simulink model "barometer"  (R2018a)
settings: Solver=VariableStepAuto  StartTime=0.0  StopTime=10.0  RelTol=1e-3
undefined symbols (not defined in the file): g
libraries: simulink_extras x1
settings Model: Creator=David  LastModifiedBy=David

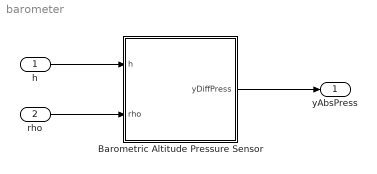
== system barometer ==
  h : Inport
  rho : Inport  Port=2
  Barometric Altitude Pressure Sensor : Subsystem  mask{SampleTime=1, absPressureNoiseDensity=0, absPressureBandwidthHz=1E06, absPressureInit=0, absPressureUpperSaturation=inf, absPressureLowerSaturation=-inf, absPressureResolution=1E-12}
      mask prompts: SampleTime "Barometric Altitude Pressure Sensor Sample Time (s)"; absPressureNoiseDensity "Barometric Altitude Pressure Sensor Noise Density (Pa/sqrt(Hz))"; absPressureBandwidthHz "Barometric Altitude Pressure Sensor Bandwidth (Hz)"; absPressureInit "Barometric Altitude Pressure Sensor Initial Condition (Pa)"; absPressureUpperSaturation "Barometric Altitude Sensor Upper Saturation Limit (Pa)"; absPressureLowerSaturation "Barometric Altitude Sensor Lower Saturation Limit (Pa)"; absPressureResolution "Barometric Altitude Pressure Sensor Resolution (Pa)"
      mask DialogControl DescGroupVar Prompt: Barometric Altitude Pressure Sensor Model
      mask DialogControl DescTextVar Prompt: Barometric Altitude Pressure Sensor with White Noise Modelling.
      mask DialogControl Control2 Prompt: If one can only get a sensor accuracy of +- error band of span, treat this as 3 sigma when calculating noise density. (ie. ((Sensor % Band)/3)*Span/(sqrt(1/SamplingTime))
      mask DialogControl Container7 Prompt: System Characteristics
      mask DialogControl Container4 Prompt: Noise Characteristics
      mask DialogControl Container6 Prompt: Sensor Dynamics
      mask DialogControl Container10 Prompt: Bandwidth
      mask DialogControl Container11 Prompt: Initial Conditions
      mask DialogControl Container8 Prompt: Limits and Quantization
      mask DialogControl Container13 Prompt: Limits
      mask DialogControl Container16 Prompt: Quantization
      mask Display:
      | image('barometer.jpg')
      | 
      | color('red')
      | 
      | port_label('input', 1, 'h (m)', 'texMode', 'on')
      | port_label('input', 2, '\rho (kg/m^3)', 'texMode', 'on')
      | 
      | port_label('output', 1, 'y_{P_{abs}} (Pa)', 'texMode', 'on')
  yAbsPress : Outport
  wires:
  h/1 -> Barometric Altitude Pressure Sensor/1(h)
  rho/1 -> Barometric Altitude Pressure Sensor/2(rho)
  Barometric Altitude Pressure Sensor/1(yDiffPress) -> yAbsPress/1

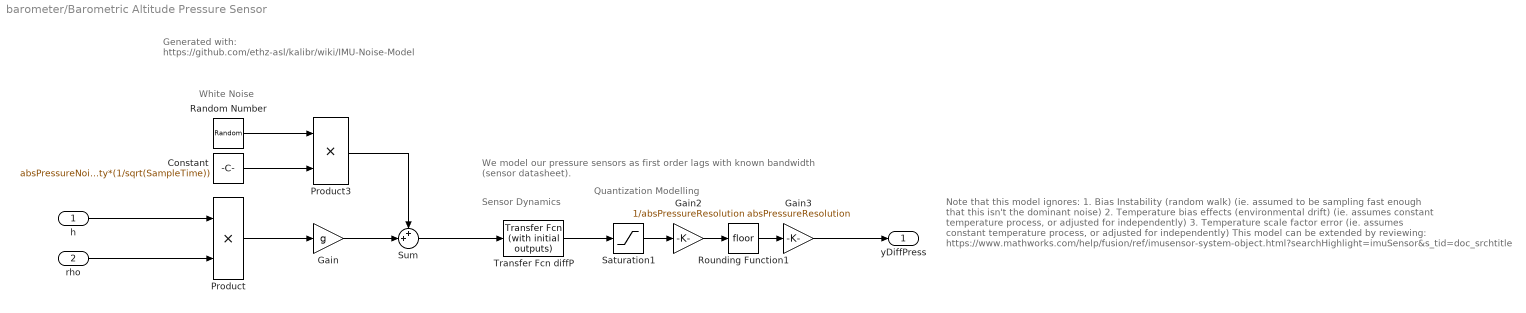
== system barometer/Barometric Altitude Pressure Sensor ==
  note: Generated with:
      | https://github.com/ethz-asl/kalibr/wiki/IMU-Noise-Model
  note: We model our pressure sensors as first order lags with known bandwidth
      | (sensor datasheet).
  note: Sensor Dynamics
  note: Quantization Modelling
  note: Note that this model ignores:
      | 1. Bias Instability (random walk) (ie. assumed to be sampling fast enough that this isn't the dominant noise)
      | 2. Temperature bias effects (environmental drift) (ie. assumes constant temperature process, or adjusted for independently)
      | 3. Temperature scale factor error (ie. assumes constant temperature process, or adjusted for independently)
      |
      | This model can be extended by reviewing:
      | https://www.mathworks.com/help/fusion/ref/imusensor-system-object.html?searchHighlight=imuSensor&s_tid=doc_srchtitle
  note: White Noise
  h : Inport
  rho : Inport  Port=2
  Constant : Constant  Value=absPressureNoiseDensity*(1/sqrt(SampleTime))
  Gain : Gain  Gain=g
  Gain2 : Gain  Gain=1/absPressureResolution
  Gain3 : Gain  Gain=absPressureResolution
  Product : Product
  Product3 : Product
  Random Number : RandomNumber  SampleTime=SampleTime
  Rounding Function1 : Rounding
  Saturation1 : Saturate  UpperLimit=absPressureUpperSaturation  LowerLimit=absPressureLowerSaturation
  Sum : Sum  Inputs=++|
  Transfer Fcn diffP : simulink_extras/Additional Linear/Transfer Fcn (with initial outputs)  N=[absPressureBandwidthHz*2*pi]  D="[1,  absPressureBandwidthHz*2*pi]"  Y0=absPressureInit  U0=absPressureInit
  yDiffPress : Outport
  wires:
  Transfer Fcn diffP/1 -> Saturation1/1
  Sum/1 -> Transfer Fcn diffP/1
  Gain2/1 -> Rounding Function1/1
  Saturation1/1 -> Gain2/1
  Gain3/1 -> yDiffPress/1
  Rounding Function1/1 -> Gain3/1
  Gain/1 -> Sum/2
  Constant/1 -> Product3/2
  Product3/1 -> Sum/1
  Product/1 -> Gain/1
  Random Number/1 -> Product3/1
  rho/1 -> Product/2
  h/1 -> Product/1
